simulink library "MEKF_Conversion_lib"  (R2018b)
settings: Solver=VariableStepAuto  StartTime=0.0  StopTime=10.0  RelTol=1e-3
undefined symbols (not defined in the file or in its folder): fswParams, simParams
libraries: maggyroProcessing_lib x2, mag_mtq_duty_cycle_lib x1, pd_processing_lib x1
settings Model: Creator=kylle  LastModifiedBy=Taylor

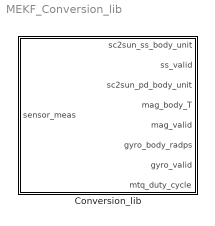
== system MEKF_Conversion_lib ==
  Conversion_lib : Subsystem

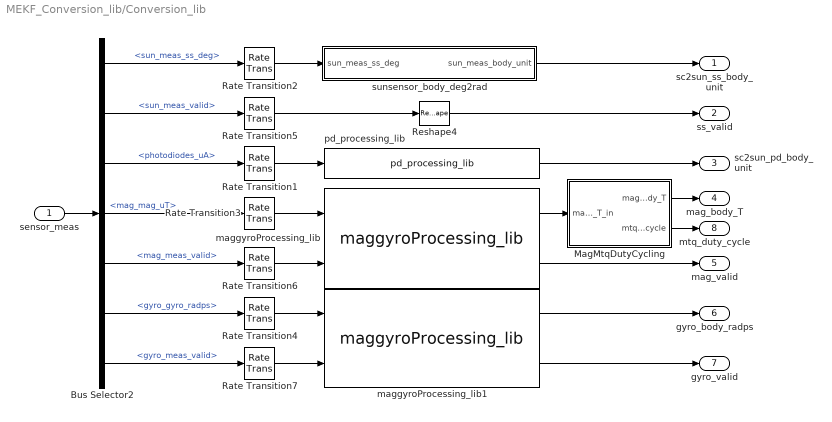
== system MEKF_Conversion_lib/Conversion_lib ==
  sensor_meas : Inport  OutDataTypeStr=Bus: sensor_bus
  Bus Selector2 : BusSelector  OutputSignals=sun_meas_ss_deg,sun_meas_valid,photodiodes_uA,mag_mag_uT,mag_meas_valid,gyro_gyro_radps,gyro_meas_valid
  MagMtqDutyCycling : Subsystem
  Rate Transition{1..7} (7 alike) : RateTransition  OutPortSampleTime=fswParams.sample_time_s
  Reshape4 : Reshape
  maggyroProcessing_lib : maggyroProcessing_lib/maggyroProcessing_lib  static_range_max_value=fswParams.sensors.mag_static_range  offset_calibration_matrix=fswParams.sensors.mag_offset  max_err=fswParams.sensors.mag_max_err  rotation_calibration_matrix=fswParams.sensors.mag_rotate  Gain=fswParams.constants.convert.uT2T
  maggyroProcessing_lib1 : maggyroProcessing_lib/maggyroProcessing_lib  static_range_max_value=fswParams.sensors.gyro_static_range  offset_calibration_matrix=fswParams.sensors.gyro_offset  max_err=fswParams.sensors.gyro_max_err  rotation_calibration_matrix=fswParams.sensors.gyro_rotate  Gain=1
  pd_processing_lib : pd_processing_lib/pd_processing_lib  SystemSampleTime=-1
  sunsensor_body_deg2rad : Subsystem
  sc2sun_ss_body_unit : Outport
  ss_valid : Outport  Port=2
  sc2sun_pd_body_unit : Outport  Port=3
  mag_body_T : Outport  Port=4
  mag_valid : Outport  Port=5
  gyro_body_radps : Outport  Port=6
  gyro_valid : Outport  Port=7
  mtq_duty_cycle : Outport  Port=8
  wires:
  Bus Selector2/2 -> Rate Transition5/1  "<sun_meas_valid>"
  sensor_meas/1 -> Bus Selector2/1
  Bus Selector2/7 -> Rate Transition7/1  "<gyro_meas_valid>"
  Bus Selector2/5 -> Rate Transition6/1  "<mag_meas_valid>"
  sunsensor_body_deg2rad/1(sun_meas_body_unit) -> sc2sun_ss_body_unit/1
  Bus Selector2/4 -> Rate Transition3/1  "<mag_mag_uT>"
  Bus Selector2/1 -> Rate Transition2/1  "<sun_meas_ss_deg>"
  Bus Selector2/6 -> Rate Transition4/1  "<gyro_gyro_radps>"
  maggyroProcessing_lib1/2 -> gyro_valid/1
  maggyroProcessing_lib/2 -> mag_valid/1
  maggyroProcessing_lib1/1 -> gyro_body_radps/1
  Reshape4/1 -> ss_valid/1
  Bus Selector2/3 -> Rate Transition1/1  "<photodiodes_uA>"
  pd_processing_lib/1 -> sc2sun_pd_body_unit/1
  Rate Transition2/1 -> sunsensor_body_deg2rad/1(sun_meas_ss_deg)
  Rate Transition1/1 -> pd_processing_lib/1
  Rate Transition3/1 -> maggyroProcessing_lib/1
  Rate Transition4/1 -> maggyroProcessing_lib1/1
  Rate Transition5/1 -> Reshape4/1
  Rate Transition6/1 -> maggyroProcessing_lib/2
  Rate Transition7/1 -> maggyroProcessing_lib1/2
  maggyroProcessing_lib/1 -> MagMtqDutyCycling/1(mag_body_T_in)
  MagMtqDutyCycling/1(mag_body_T) -> mag_body_T/1
  MagMtqDutyCycling/2(mtq_duty_cycle) -> mtq_duty_cycle/1

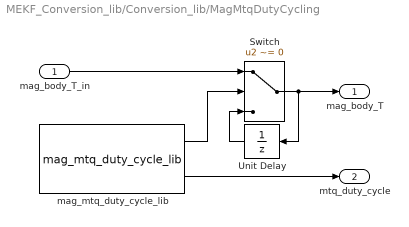
== system MEKF_Conversion_lib/Conversion_lib/MagMtqDutyCycling ==
  mag_body_T_in : Inport
  Switch : Switch  Criteria=u2 ~= 0  OutDataTypeStr=double  InputSameDT=on
  Unit Delay : UnitDelay  InitialCondition=[0;0;1]  SampleTime=-1
  mag_mtq_duty_cycle_lib : mag_mtq_duty_cycle_lib/mag_mtq_duty_cycle_lib  SystemSampleTime=-1
  mag_body_T : Outport
  mtq_duty_cycle : Outport  Port=2
  wires:
  mag_mtq_duty_cycle_lib/1 -> Switch/2
  mag_mtq_duty_cycle_lib/2 -> mtq_duty_cycle/1
  mag_body_T_in/1 -> Switch/1
  Unit Delay/1 -> Switch/3
  Switch/1 -> Unit Delay/1, mag_body_T/1

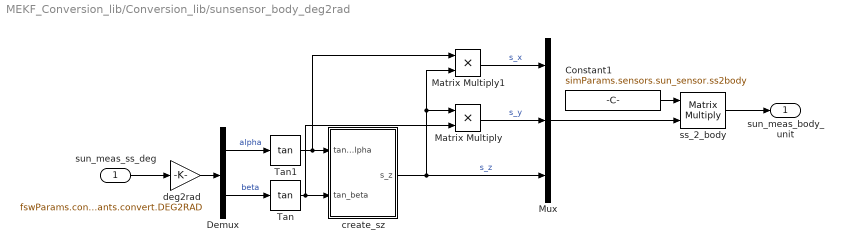
== system MEKF_Conversion_lib/Conversion_lib/sunsensor_body_deg2rad ==
  sun_meas_ss_deg : Inport
  Constant1 : Constant  Value=simParams.sensors.sun_sensor.ss2body
  Demux : Demux  Outputs=2
  Matrix Multiply : Product
  Matrix Multiply1 : Product
  Mux : Mux  Inputs=3
  Tan : Trigonometry  Operator=tan
  Tan1 : Trigonometry  Operator=tan
  create_sz : Subsystem
  deg2rad : Gain  Gain=fswParams.constants.convert.DEG2RAD
  ss_2_body : Product  Multiplication=Matrix(*)
  sun_meas_body_unit : Outport
  wires:
  create_sz/1(s_z) -> Matrix Multiply/1, Matrix Multiply1/2, Mux/3  "s_z"
  Matrix Multiply1/1 -> Mux/1  "s_x"
  ss_2_body/1 -> sun_meas_body_unit/1
  Mux/1 -> ss_2_body/2
  Constant1/1 -> ss_2_body/1
  sun_meas_ss_deg/1 -> deg2rad/1
  deg2rad/1 -> Demux/1
  Demux/2 -> Tan/1  "beta"
  Demux/1 -> Tan1/1  "alpha"
  Tan1/1 -> Matrix Multiply1/1, create_sz/1(tan_alpha)
  Tan/1 -> Matrix Multiply/2, create_sz/2(tan_beta)
  Matrix Multiply/1 -> Mux/2  "s_y"

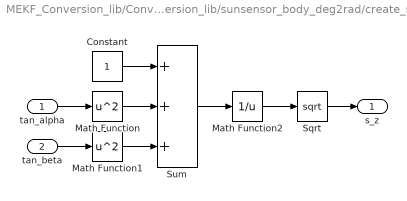
== system MEKF_Conversion_lib/Conversion_lib/sunsensor_body_deg2rad/create_sz ==
  tan_alpha : Inport
  tan_beta : Inport  Port=2
  Constant : Constant
  Math Function : Math  Operator=square  SaturateOnIntegerOverflow=on
  Math Function1 : Math  Operator=square  SaturateOnIntegerOverflow=on
  Math Function2 : Math  Operator=reciprocal  SaturateOnIntegerOverflow=on
  Sqrt : Sqrt  SaturateOnIntegerOverflow=on
  Sum : Sum  Inputs=+++
  s_z : Outport
  wires:
  Sqrt/1 -> s_z/1
  Math Function1/1 -> Sum/3
  tan_beta/1 -> Math Function1/1
  Math Function2/1 -> Sqrt/1
  Math Function/1 -> Sum/2
  tan_alpha/1 -> Math Function/1
  Sum/1 -> Math Function2/1
  Constant/1 -> Sum/1
